simulink model "test"  (R2023b)
settings: Solver=VariableStepAuto  StartTime=0.0  StopTime=200  RelTol=1e-3
undefined symbols (not defined in the file or in its folder): env, init, X8
libraries: Fixed_Wing x5
settings Model: Creator=NCS  LastModifiedBy=NCS

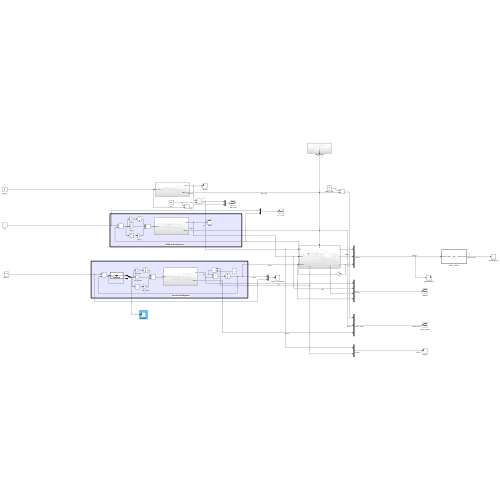
[thumbnail: Simulink's stored preview of the top-level diagram]
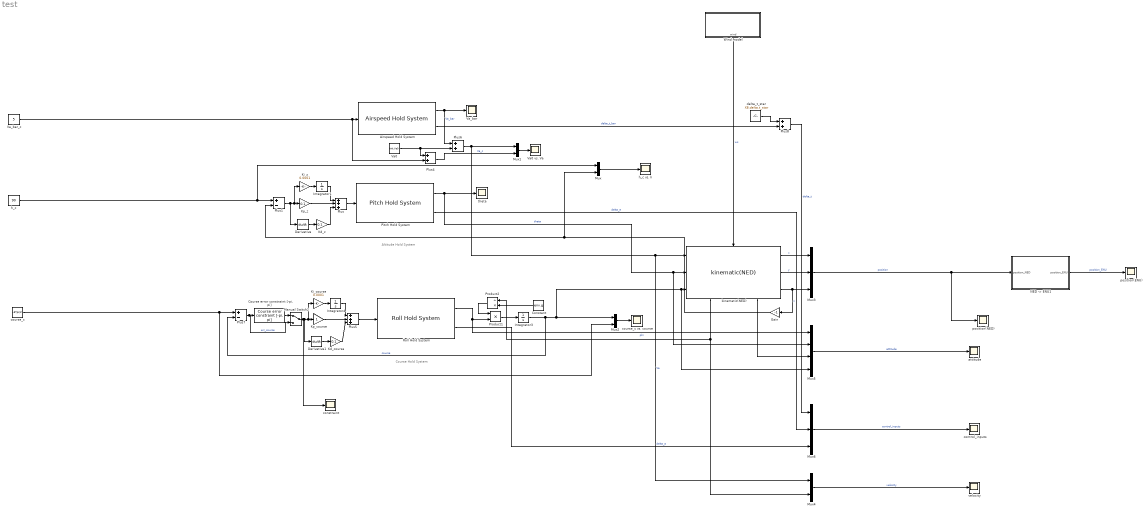
== system test ==
  note: Course Hold System
  note: Altitude Hold System
  Airspeed Hold System : Fixed_Wing/Airspeed Hold System  SystemSampleTime=-1  VariantActivationTime=update diagram  AllowFlexibleInterface=on  Latency=0  AutoFrameSizeCalculation=off
      settings: SourceProductName=Fixed-Wing Model
  Constant : Constant  Value=env.g
  "Course error constraint [-pi, pi]" : Fixed_Wing/Fixed Wing Model/Course error constraint [-pi, pi]  SystemSampleTime=-1  VariantActivationTime=update diagram  AllowFlexibleInterface=on  Latency=0  AutoFrameSizeCalculation=off
      settings: SourceProductName=Fixed-Wing Model
  Derivative : Derivative
  Derivative1 : Derivative
  Gain : Gain  Gain=-1
  Integrator1 : Integrator
  Integrator3 : Integrator  InitialCondition=init.course0
  Integrator4 : Integrator
  Kd_course : Gain  Gain=0.1
  Kd_z : Gain  Gain=0.1
  Ki_course : Gain  Gain=0.0001
  Ki_z : Gain  Gain=0.0001
  Kp_course : Gain
  Kp_z : Gain  Gain=0.1
  Manual Switch2 : ManualSwitch
  Mux{,1..2,4} (4 alike) : Mux  Inputs=2
  Mux3 : Mux  Inputs=3
  Mux5 : Mux
  Mux6 : Mux  Inputs=3
  "NED -> ENU1" : MATLAB Function  TreatAsAtomicUnit=on
  "Pitch Hold System " : Fixed_Wing/Pitch Hold System   SystemSampleTime=-1  VariantActivationTime=update diagram  AllowFlexibleInterface=on  Latency=0  AutoFrameSizeCalculation=off
      settings: SourceProductName=Fixed-Wing Model
  Plus : Sum  Inputs=+++
  Plus1 : Sum  Inputs=+-
  Plus4 : Sum
  Plus5 : Sum  Inputs=+++
  Plus6 : Sum
  Plus7 : Sum  Inputs=+-
  Plus8 : Sum
  Product1 : Product
  Product2 : Product  Inputs=/*
  Roll Hold System : Fixed_Wing/Roll Hold System  SystemSampleTime=-1  VariantActivationTime=update diagram  AllowFlexibleInterface=on  Latency=0  AutoFrameSizeCalculation=off
      settings: SourceProductName=Fixed-Wing Model
  Va0 : Constant  Value=init.Va0
  Va0 vs. Va : Scope
  Va_bar : Scope
  Va_bar_c : Constant  Value=5
  Wind model : Subsystem
      settings: PortSchema="{\"entries\":[{\"content\":{\"sides\":[{\"content\":{},\"type\":\"ConnectorPlacement.EquallySpacedRectSide\",\"uuid\":\"19ef0eb7-c626-45ec-b76b-8668fc024824\"},{\"content\":{\"side\":\"RIGHT\"},\"type\":\"ConnectorPlacement.EquallySpacedRectSide\",\"uuid\":\"89e72569-ab94-4162-a6e2-b425ef08f724\"},{\"content\":{\"side\":\"TOP\"},\"type\":\"ConnectorPlacement.EquallySpacedRectSide\",\"uuid\":\"6d9409e9-6822-4cd9-902f-e5665cb68433\"},{\"content\":{\"connectorIds\":[\"Out1\"],\"side\":\"BOTTOM\"},\"type\":\"ConnectorPlacement.EquallySpacedRectSide\",\"uuid\":\"39a83352-0924-44fa-be5d-94a7c28bbbf3\"}]},\"type\":\"ConnectorPlacement.EquallySpacedConnector\",\"uuid\":\"6cf6ae00-ef23-42a2-99b2-ca60e191fb03\"}],\"packageUris\":[\"http://schema.mathworks.com/mf0/Connector/R2020b\"],\"version\":\"1.0\"}"
  attitude : Scope
  constraint : Scope
  control_inputs : Scope
  course_c : Constant  Value=-3*pi/2
  course_c vs. course : Scope
  delta_t_star : Constant  Value=X8.delta.t_star
  h_c : Constant  Value=90
  h_c vs. h : Scope
  kinematic(NED) : Fixed_Wing/kinematic(NED)  SystemSampleTime=-1  VariantActivationTime=update diagram  AllowFlexibleInterface=on  Latency=0  AutoFrameSizeCalculation=off
      settings: SourceProductName=Fixed-Wing Model  PortSchema="{\"entries\":[{\"content\":{\"sides\":[{\"content\":{\"connectorIds\":[\"In1\",\"In2\",\"In3\"]},\"type\":\"ConnectorPlacement.EquallySpacedRectSide\",\"uuid\":\"96d967d8-b822-4ab1-b08a-27adc20d5833\"},{\"content\":{\"connectorIds\":[\"Out1\",\"Out2\",\"Out3\"],\"side\":\"RIGHT\"},\"type\":\"ConnectorPlacement.EquallySpacedRectSide\",\"uuid\":\"505a36c9-cae2-422c-97bf-34d37872a31d\"},{\"content\":{\"connectorIds\":[\"In4\"],\"side\":\"TOP\"},\"type\":\"ConnectorPlacement.EquallySpacedRectSide\",\"uuid\":\"7bc53155-5df6-4b6a-9756-725497693b0a\"},{\"content\":{\"connectorIds\":[\"Out4\",\"Out5\"],\"side\":\"BOTTOM\"},\"type\":\"ConnectorPlacement.EquallySpacedRectSide\",\"uuid\":\"7777b465-a27e-4b61-9b89-f3b8fa4654d1\"}]},\"type\":\"ConnectorPlacement.EquallySpacedConnector\",\"uuid\":\"2150a812-5a4a-4a29-9c93-d226d95b2326\"}],\"packageUris\":[\"http://schema.mathworks.com/mf0/Connector/R2020b\"],\"version\":\"1.0\"}"
  position(ENU) : Scope
  position(NED) : Scope
  theta : Scope
  velocity : Scope
  wires:
  Mux4/1 -> velocity/1  "velocity"
  Mux3/1 -> position(NED)/1, "NED -> ENU1"/1(position_NED)  "position"
  "NED -> ENU1"/1(position_ENU) -> position(ENU)/1  "position_ENU"
  Mux6/1 -> control_inputs/1  "control_inputs"
  Mux2/1 -> course_c vs. course/1
  Roll Hold System/2 -> Mux6/3  "delta_a"
  kinematic(NED)/5 -> Mux5/3
  Plus/1 -> "Pitch Hold System "/1
  Integrator1/1 -> Plus/1
  kinematic(NED)/3 -> Mux3/3, Gain/1  "z"
  Integrator4/1 -> Plus5/1
  "Pitch Hold System "/1 -> theta/1, Mux5/2, kinematic(NED)/2  "theta"
  Airspeed Hold System/1 -> Va_bar/1, Plus6/1  "Va_bar"
  Gain/1 -> Plus1/2, Mux/2
  Kd_z/1 -> Plus/3
  Derivative1/1 -> Kd_course/1
  kinematic(NED)/1 -> Mux3/1  "x"
  Constant/1 -> Product2/2
  kinematic(NED)/4 -> Product2/1, Mux4/2
  kinematic(NED)/2 -> Mux3/2  "y"
  Plus1/1 -> Kp_z/1, Ki_z/1, Derivative/1
  Integrator3/1 -> Plus7/2, Mux2/1, kinematic(NED)/3, Mux5/4  "course"
  Derivative/1 -> Kd_z/1
  Va0/1 -> Plus6/2, Plus4/1
  Plus8/1 -> Mux6/1  "delta_t"
  delta_t_star/1 -> Plus8/1
  Kp_z/1 -> Plus/2
  Airspeed Hold System/2 -> Plus8/2  "delta_t_bar"
  course_c/1 -> Plus7/1, Mux2/2
  Plus6/1 -> Mux4/1, kinematic(NED)/1, Mux1/1  "Va"
  "Pitch Hold System "/2 -> Mux6/2  "delta_e"
  Va_bar_c/1 -> Airspeed Hold System/1, Plus4/2
  Mux/1 -> h_c vs. h/1
  Product2/1 -> Product1/1
  Plus7/1 -> "Course error constraint [-pi, pi]"/1, Manual Switch2/2  "err_course"
  Kd_course/1 -> Plus5/3
  h_c/1 -> Plus1/1, Mux/1
  Plus4/1 -> Mux1/2  "Va_c"
  Mux1/1 -> Va0 vs. Va/1
  Ki_course/1 -> Integrator4/1
  Roll Hold System/1 -> Product1/2, Mux5/1  "phi"
  Manual Switch2/1 -> constraint/1, Kp_course/1, Ki_course/1, Derivative1/1
  "Course error constraint [-pi, pi]"/1 -> Manual Switch2/1
  Kp_course/1 -> Plus5/2
  Plus5/1 -> Roll Hold System/1
  Ki_z/1 -> Integrator1/1
  Product1/1 -> Integrator3/1
  Wind model/1(wind) -> kinematic(NED)/4  "ws"
  Mux5/1 -> attitude/1  "attitude"

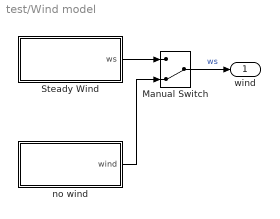
== system test/Wind model ==
  Manual Switch : ManualSwitch  CurrentSetting=0
  "Steady Wind " : Subsystem
  no wind : Subsystem
  wind : Outport
  wires:
  "Steady Wind "/1(ws) -> Manual Switch/1
  no wind/1(wind) -> Manual Switch/2
  Manual Switch/1 -> wind/1  "ws"

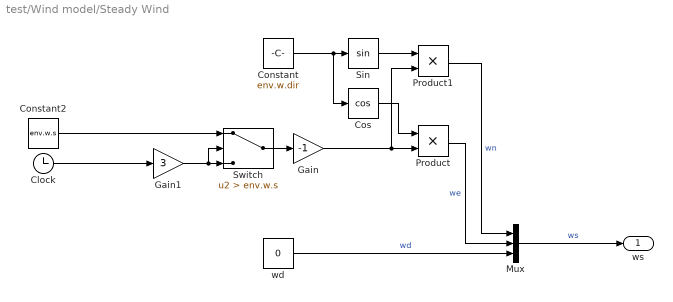
== system test/Wind model/Steady Wind  ==
  Clock : Clock
  Constant : Constant  Value=env.w.dir
  Constant2 : Constant  Value=env.w.s
  Cos : Trigonometry  Operator=cos
  Gain : Gain  Gain=-1
  Gain1 : Gain  Gain=3
  Mux : Mux  Inputs=3
  Product : Product
  Product1 : Product
  Sin : Trigonometry
  Switch : Switch  Criteria=u2 > Threshold  Threshold=env.w.s  SaturateOnIntegerOverflow=off  InputSameDT=off
  wd : Constant  Value=0
  ws : Outport
  wires:
  wd/1 -> Mux/3  "wd"
  Mux/1 -> ws/1  "ws"
  Product1/1 -> Mux/1  "wn"
  Product/1 -> Mux/2  "we"
  Constant/1 -> Cos/1, Sin/1
  Cos/1 -> Product/1
  Sin/1 -> Product1/1
  Gain/1 -> Product1/2, Product/2
  Clock/1 -> Gain1/1
  Gain1/1 -> Switch/2, Switch/3
  Constant2/1 -> Switch/1
  Switch/1 -> Gain/1

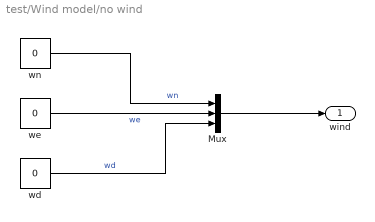
== system test/Wind model/no wind ==
  Mux : Mux  Inputs=3
  wd : Constant  Value=0
  we : Constant  Value=0
  wn : Constant  Value=0
  wind : Outport
  wires:
  wd/1 -> Mux/3  "wd"
  Mux/1 -> wind/1
  wn/1 -> Mux/1  "wn"
  we/1 -> Mux/2  "we"

== matlab function test/NED -> ENU1 ==
  data: position_NED input; position_ENU output
function position_ENU = fcn(position_NED)
R_NED_ENU = [0 1 0;
             1 0 0;
             0 0 -1;];
position_ENU = R_NED_ENU* position_NED;
end
